simulink model "HybridStationAcceptanceTest_r1"  (R2023a)
settings: Solver=VariableStepAuto  StartTime=0.0  StopTime=240  RelTol=1e-3
libraries: simulink x43, simulink_extras x12, dspswit3 x10, spspowerguiLib x1
settings Model: PacingRate=4  Creator=jakob  LastModifiedBy=matty

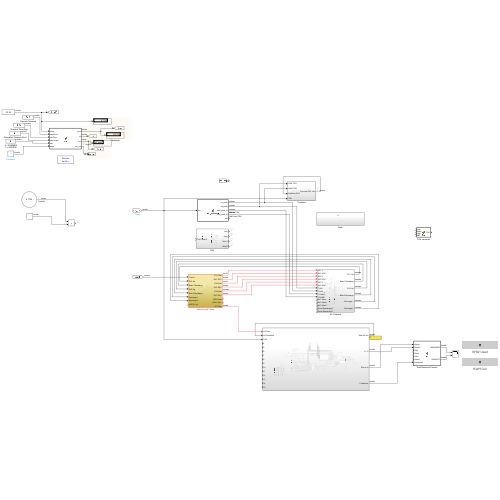
[thumbnail: Simulink's stored preview of the top-level diagram]
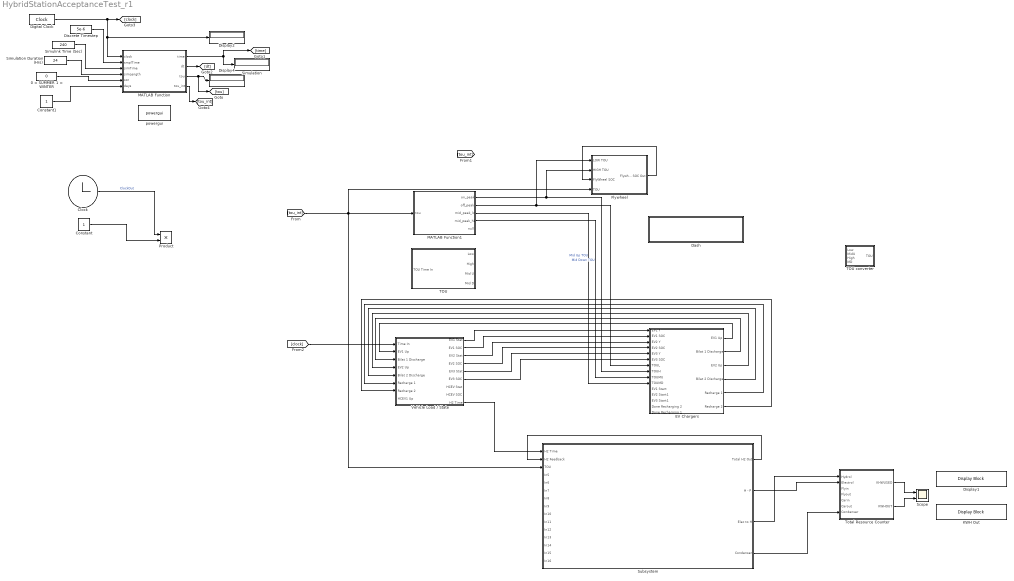
== system HybridStationAcceptanceTest_r1 ==
  0 = SUMMER 1 = WINTER : Constant  Value=0
  Clock : Clock
  Constant : Constant
  Constant1 : Constant
  Dash : Subsystem
  Digital Clock : DigitalClock  SampleTime=5e-6
  Discrete Timestep : Constant  Value=5e-6
  Display1 : DisplayBlock  LabelPosition=Hide  Transparency=1
      settings: AttributesFormatString=KHW Used
  Display2 : Display
  Display4 : Display
  EV Chargers : Subsystem
  Flywheel : Subsystem  StopFcn=CapTest
  KWH Out : DisplayBlock  LabelPosition=Hide  Transparency=1
      settings: AttributesFormatString=KWH Out
  MATLAB Function : MATLAB Function  TreatAsAtomicUnit=on
  MATLAB Function1 : MATLAB Function  TreatAsAtomicUnit=on
  Product : Product
  Scope : Scope  NumInputPorts=2
  Simulation : Display
  Simulation Duration (Hrs) : Constant  Value=24
  Simulink Time (Sec) : Constant  Value=240
  Subsystem : Subsystem
  TOU : Subsystem
  TOU converter : MATLAB Function  TreatAsAtomicUnit=on
  Total Resource Counter : MATLAB Function  TreatAsAtomicUnit=on
  Vehicle Load / State : Subsystem
  powergui : spspowerguiLib/powergui  Priority=1  SimulationMode=Discrete  SampleTime=5e-6  frequency=60  Iterations=50  frequencyindice=0  Pbase=100e6  ErrMax=1e-4  UnitsV=kV  UnitsW=MW  buscounter=0  FunctionMessages=off  echomessages=off  EnableUseOfTLC=off  CurrentSourceSwitches=off  DisableSnubberDevices=off  DisableRonSwitches=off  DisableVfSwitches=off  DisplayEquations=off  AutomaticDiscreteSolvers=off  SolverType=Tustin/Backward Euler (TBE)  Interpol=off  ExternalGateDelay=off  methode=off  Ts=100  x0status=blocks  SPID=on  SwTol=0  HookPort=off  NonlinearTolerance=1e-4  nMaxIteration=100  ContinueOnMaxIteration=off  RestoreLinks=warning  ResistiveCurrentMeasurement=off  Frange=[0:2:500]  Ylog=off  Xlog=on  ShowGrid=off  save=off  variable=ZData  structure=0  ZoomFFT=off  StartTime=0.0  cycles=1  DisplayStyle=1  fundamental=60  FreqAxis=off  MaxFrequency=1000  frequencyindicesteady=1  RmsSteady=1  display=off
  wires:
  Clock/1 -> Product/1  "ClockOut"
  Constant/1 -> Product/2
  Vehicle Load / State/1(EV1 Stat) -> EV Chargers/1(EV1 Y)
  Vehicle Load / State/2(EV1 SOC) -> EV Chargers/2(EV1 SOC)
  Vehicle Load / State/3(EV2 Stat) -> EV Chargers/3(EV2 Y)
  Vehicle Load / State/4(EV2 SOC) -> EV Chargers/4(EV2 SOC)
  Vehicle Load / State/5(EV3 Stat) -> EV Chargers/5(EV3 Y)
  Vehicle Load / State/6(EV3 SOC) -> EV Chargers/6(EV3 SOC)
  Flywheel/1(Flywheel SOC Out) -> Flywheel/3(FlyWheel SOC)
  EV Chargers/1(EV1 Up) -> Vehicle Load / State/2(EV1 Up)
  EV Chargers/2(Bilat 1 Discharge) -> Vehicle Load / State/3(Bilat 1 Discharge)
  EV Chargers/3(EV2 Up) -> Vehicle Load / State/4(EV2 Up)
  EV Chargers/4(Bilat 2 Discharge) -> Vehicle Load / State/5(Bilat 2 Discharge)
  EV Chargers/5(Recharge 1) -> Vehicle Load / State/6(Recharge 1)
  EV Chargers/6(Recharge 2) -> Vehicle Load / State/7(Recharge 2)
  Vehicle Load / State/9(H2 Time) -> Subsystem/1(H2 Time)
  Subsystem/1(Total H2 Out) -> Subsystem/2(H2 Feedback)
  Total Resource Counter/1(KHWUSED) -> Scope/1
  Total Resource Counter/2(KWHOUT) -> Scope/2
  Subsystem/4(Condenser) -> Total Resource Counter/7(Condenser)
  Subsystem/3(Elec to H) -> Total Resource Counter/1(Hydrol)
  Subsystem/2(H - P) -> Total Resource Counter/2(Electrol)
  MATLAB Function/1(time) -> [time], Simulation/1
  MATLAB Function/3(tou) -> [tou], Display4/1
  Digital Clock/1 -> [clock], MATLAB Function/1(clock), Display2/1
  Constant1/1 -> MATLAB Function/6(days)
  Discrete Timestep/1 -> MATLAB Function/2(smplTime)
  Simulink Time (Sec)/1 -> MATLAB Function/3(simTime)
  Simulation Duration (Hrs)/1 -> MATLAB Function/4(simLength)
  MATLAB Function/4(tou_int) -> [tou_int]
  MATLAB Function/2(dt) -> [dt]
  0 = SUMMER 1 = WINTER/1 -> MATLAB Function/5(szn)
  [tou_int] -> Subsystem/3(TOU), Flywheel/4(TOU), MATLAB Function1/1(tou)
  MATLAB Function1/3(mid_peak_lo) -> EV Chargers/10(TOUMD)  "Mid Up TOU"
  MATLAB Function1/1(on_peak) -> Flywheel/2(HIGH TOU), EV Chargers/8(TOUH)
  MATLAB Function1/2(off_peak) -> Flywheel/1(LOW TOU), EV Chargers/7(TOUL)
  MATLAB Function1/4(mid_peak_hi) -> EV Chargers/9(TOUMU)  "Mid Down TOU"
  [clock] -> Vehicle Load / State/1(Time In)

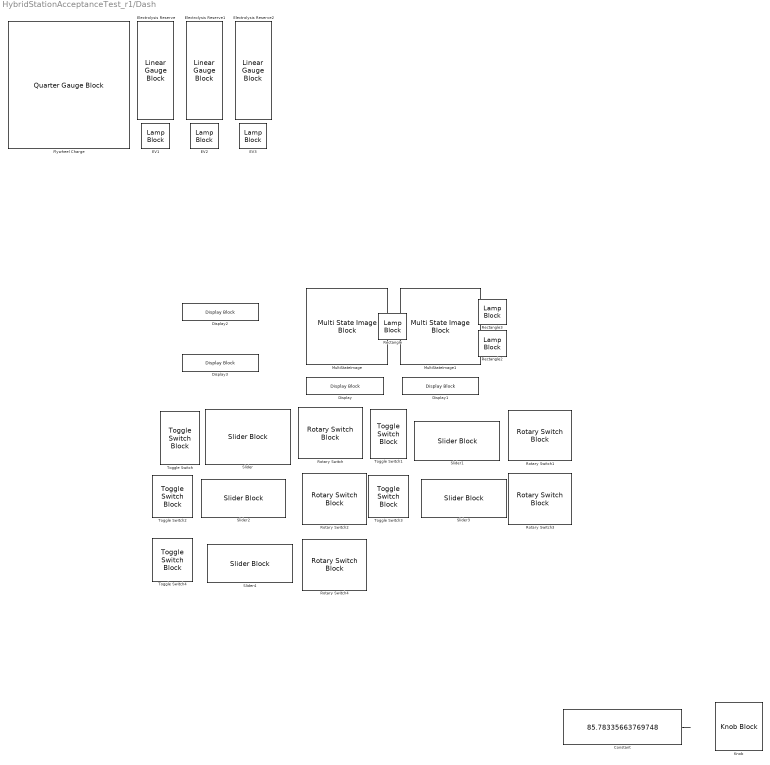
== system HybridStationAcceptanceTest_r1/Dash ==
  Constant : Constant  Value=85.78335663769748
  Display{,1..3} (4 alike) : DisplayBlock  LabelPosition=Hide  Transparency=1
      Display2 settings: AttributesFormatString=Hydrogen Output (KG)
      Display3 settings: AttributesFormatString=FCEVs Fueled
  EV1 : LampBlock  LabelPosition=Hide
  EV2 : LampBlock  LabelPosition=Hide
  EV3 : LampBlock  LabelPosition=Hide
  Electrolysis Reserve : LinearGaugeBlock  Tag=Flywheel %
  Electrolysis Reserve1 : LinearGaugeBlock  Tag=Flywheel %
  Electrolysis Reserve2 : LinearGaugeBlock  Tag=Flywheel %
  Flywheel Charge : QuarterGaugeBlock
  Knob : KnobBlock  ScaleMax=240
  MultiStateImage : MultiStateImageBlock  Description=10KG pressurized 700Bar
      settings: AttributesFormatString=10KG pressurized 700Bar
  MultiStateImage1 : MultiStateImageBlock
      settings: AttributesFormatString=10KG pressurized 200Bar
  Rectangle : LampBlock  LabelPosition=Hide  Icon=Rectangle
      settings: AttributesFormatString=Compressor
  Rectangle2 : LampBlock  LabelPosition=Hide  Icon=Rectangle
      settings: AttributesFormatString=Reverse Electrolysis
  Rectangle3 : LampBlock  LabelPosition=Hide  Icon=Rectangle
      settings: AttributesFormatString=Electrolysis
  Rotary Switch{,1..4} (5 alike) : RotarySwitchBlock
      settings: Values={{'>0', '1', '2', '3', '4'}, [0 1 2 3 4]}
      settings: AttributesFormatString=Hydrogren Level
  Slider{,1..4} (5 alike) : SliderBlock  ScaleMax=240
      settings: AttributesFormatString=Start Time
  Toggle Switch{,1..4} (5 alike) : ToggleSwitchBlock
      settings: Values={{'Off', 'On'}, [0 1]}
  wires:
  Constant/1 -> ?

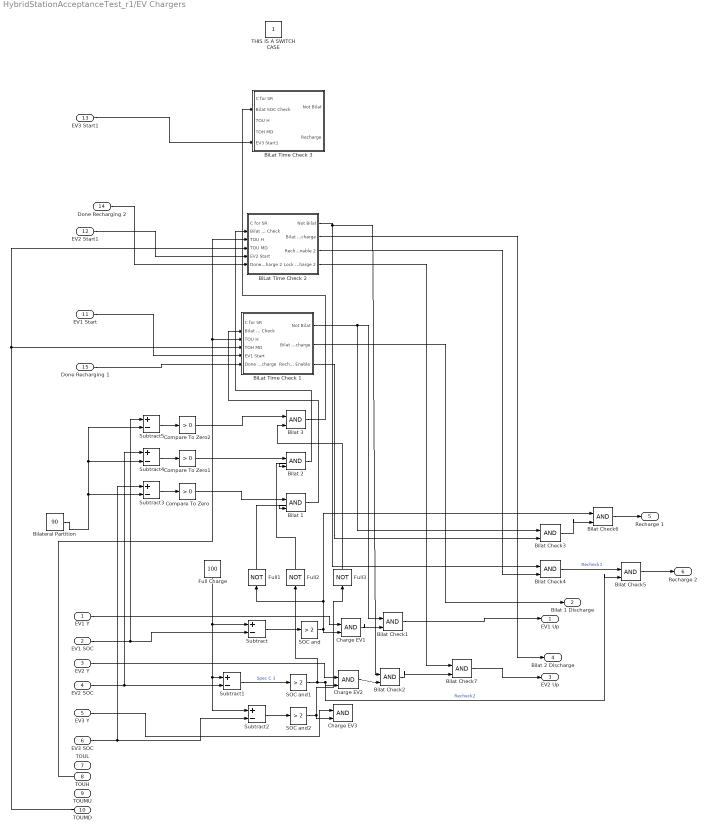
== system HybridStationAcceptanceTest_r1/EV Chargers ==
  EV1 Y : Inport
  EV1 SOC : Inport  Port=2
  EV2 Y : Inport  Port=3
  EV2 SOC : Inport  Port=4
  EV3 Y : Inport  Port=5
  EV3 SOC : Inport  Port=6
  TOUL : Inport  Port=7
  TOUH : Inport  Port=8
  TOUMU : Inport  Port=9
  TOUMD : Inport  Port=10
  EV1 Start : Inport  Port=11
  EV2 Start1 : Inport  Port=12
  EV3 Start1 : Inport  Port=13
  Done Recharging 2 : Inport  Port=14
  Done Recharging 1 : Inport  Port=15
  BiLat Time Check 1 : Subsystem
  BiLat Time Check 2 : Subsystem
  BiLat Time Check 3 : Subsystem
  Bilat 1 : Logic  IconShape=distinctive  AllPortsSameDT=off  OutDataTypeStr=boolean
  Bilat 2 : Logic  IconShape=distinctive  AllPortsSameDT=off  OutDataTypeStr=boolean
  Bilat 3 : Logic  IconShape=distinctive  AllPortsSameDT=off  OutDataTypeStr=boolean
  Bilat Check{1..7} (7 alike) : Logic  IconShape=distinctive  AllPortsSameDT=off  OutDataTypeStr=boolean
  Bilateral Partition : Constant  Value=90
  Charge EV1 : Logic  IconShape=distinctive  AllPortsSameDT=off  OutDataTypeStr=boolean
  Charge EV2 : Logic  IconShape=distinctive  AllPortsSameDT=off  OutDataTypeStr=boolean
  Charge EV3 : Logic  IconShape=distinctive  AllPortsSameDT=off  OutDataTypeStr=boolean
  Compare To Zero : simulink/Logic and Bit Operations/Compare To Zero  relop=>  OutDataTypeStr=boolean
  Compare To Zero1 : simulink/Logic and Bit Operations/Compare To Zero  relop=>  OutDataTypeStr=boolean
  Compare To Zero2 : simulink/Logic and Bit Operations/Compare To Zero  relop=>  OutDataTypeStr=boolean
  Full Charge : Constant  Value=100
  Full1 : Logic  Operator=NOT  IconShape=distinctive  AllPortsSameDT=off  OutDataTypeStr=boolean
  Full2 : Logic  Operator=NOT  IconShape=distinctive  AllPortsSameDT=off  OutDataTypeStr=boolean
  Full3 : Logic  Operator=NOT  IconShape=distinctive  AllPortsSameDT=off  OutDataTypeStr=boolean
  SOC and : simulink/Logic and Bit Operations/Compare To Constant  relop=>  const=2  OutDataTypeStr=boolean
  SOC and1 : simulink/Logic and Bit Operations/Compare To Constant  relop=>  const=2  OutDataTypeStr=boolean
  SOC and2 : simulink/Logic and Bit Operations/Compare To Constant  relop=>  const=2  OutDataTypeStr=boolean
  Subtract{,1..5} (6 alike) : Sum  Inputs=+-
  THIS IS A SWITCH CASE : Constant
  EV1 Up : Outport
  Bilat 1 Discharge : Outport  Port=2
  EV2 Up : Outport  Port=3
  Bilat 2 Discharge : Outport  Port=4
  Recharge 1 : Outport  Port=5
  Recharge 2 : Outport  Port=6
  wires:
  Full Charge/1 -> Subtract2/1, Subtract1/1, Subtract/1
  EV1 SOC/1 -> Subtract5/1, Subtract/2
  EV2 Y/1 -> Charge EV2/1
  SOC and1/1 -> Bilat Check5/2, Charge EV2/2, Full2/1  "Recheck2"
  Subtract1/1 -> SOC and1/1  "Spec C 3"
  SOC and2/1 -> Full3/1, Charge EV3/2
  SOC and/1 -> Bilat Check6/1, Full1/1, Charge EV1/2
  Subtract/1 -> SOC and/1
  Subtract2/1 -> SOC and2/1
  EV3 SOC/1 -> Subtract3/1, Subtract2/2
  Charge EV2/1 -> Bilat Check2/2
  EV1 Y/1 -> Charge EV1/1
  EV3 Y/1 -> Charge EV3/1
  EV2 SOC/1 -> Subtract4/1, Subtract1/2
  Subtract3/1 -> Compare To Zero/1
  Subtract4/1 -> Compare To Zero1/1
  Subtract5/1 -> Compare To Zero2/1
  Full1/1 -> Bilat 1/2
  Compare To Zero/1 -> Bilat 1/1
  Compare To Zero1/1 -> Bilat 2/1
  Compare To Zero2/1 -> Bilat 3/1
  Full2/1 -> Bilat 2/2
  Full3/1 -> Bilat 3/2
  Bilateral Partition/1 -> Subtract4/2, Subtract5/2, Subtract3/2
  Bilat 3/1 -> BiLat Time Check 3/2(Bilat SOC Check)
  Bilat 2/1 -> BiLat Time Check 2/2(Bilat SOC Check)
  EV1 Start/1 -> BiLat Time Check 1/5(EV1 Start)
  Bilat 1/1 -> BiLat Time Check 1/2(Bilat SOC Check)
  TOUH/1 -> BiLat Time Check 2/3(TOU H), BiLat Time Check 1/3(TOU H)
  TOUMD/1 -> BiLat Time Check 2/4(TOU MD), BiLat Time Check 1/4(TOH MD)
  BiLat Time Check 1/2(Bilat Discharge) -> Bilat 1 Discharge/1
  BiLat Time Check 1/1(Not Bilat) -> Bilat Check3/1, Bilat Check1/1
  Charge EV1/1 -> Bilat Check1/2
  EV2 Start1/1 -> BiLat Time Check 2/5(EV2 Start)
  EV3 Start1/1 -> BiLat Time Check 3/5(EV3 Start1)
  BiLat Time Check 2/1(Not Bilat) -> Bilat Check4/1, Bilat Check2/1
  BiLat Time Check 2/2(Bilat Discharge) -> Bilat 2 Discharge/1
  Bilat Check2/1 -> Bilat Check7/2
  Bilat Check1/1 -> EV1 Up/1
  BiLat Time Check 1/3(Recharge Enable) -> Bilat Check3/2
  BiLat Time Check 2/3(Recharge Enable 2) -> Bilat Check4/2
  Done Recharging 2/1 -> BiLat Time Check 2/6(Done Recharge 2)
  Done Recharging 1/1 -> BiLat Time Check 1/6(Done Recharge)
  Bilat Check3/1 -> Bilat Check6/2
  Bilat Check4/1 -> Bilat Check5/1  "Recheck1"
  Bilat Check5/1 -> Recharge 2/1
  Bilat Check6/1 -> Recharge 1/1
  Bilat Check7/1 -> EV2 Up/1
  BiLat Time Check 2/4(Lock Out Recharge 2) -> Bilat Check7/1

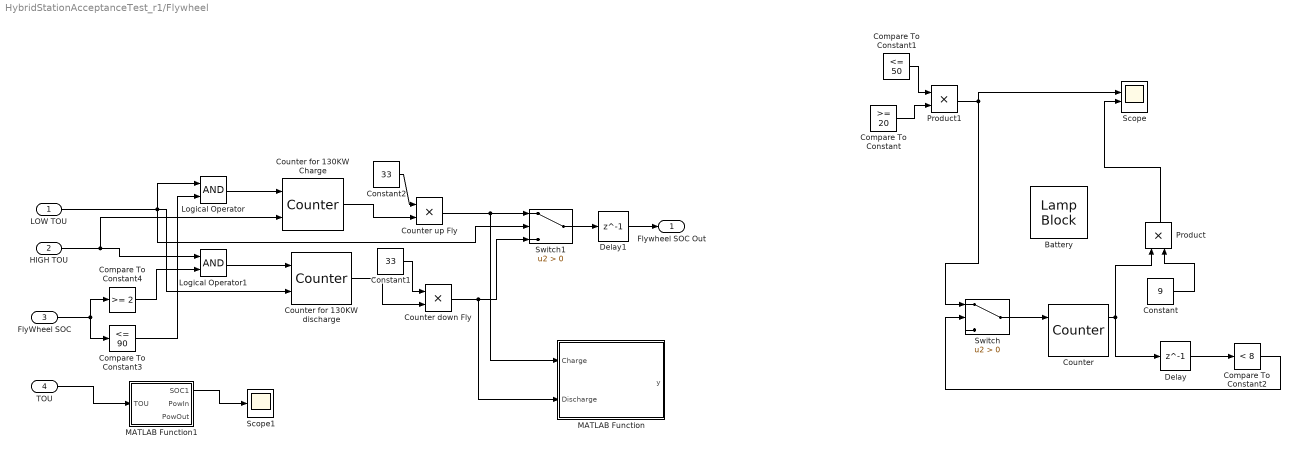
== system HybridStationAcceptanceTest_r1/Flywheel ==
  LOW TOU : Inport
  HIGH TOU : Inport  Port=2
  FlyWheel SOC : Inport  Port=3
  TOU : Inport  Port=4
  Battery : LampBlock  LabelPosition=Hide  Icon=Battery
  Compare To Constant : simulink/Logic and Bit Operations/Compare To Constant  relop=>=  const=20  OutDataTypeStr=boolean
  Compare To Constant1 : simulink/Logic and Bit Operations/Compare To Constant  relop=<=  const=50  OutDataTypeStr=boolean
  Compare To Constant2 : simulink/Logic and Bit Operations/Compare To Constant  relop=<  const=8  OutDataTypeStr=boolean
  Compare To Constant3 : simulink/Logic and Bit Operations/Compare To Constant  relop=<=  const=90  OutDataTypeStr=boolean
  Compare To Constant4 : simulink/Logic and Bit Operations/Compare To Constant  relop=>=  const=2  OutDataTypeStr=boolean
  Constant : Constant  Value=9
  Constant1 : Constant  Value=33
  Constant2 : Constant  Value=33
  Counter : dspswit3/Counter  Direction=Up  CountEvent=Non-zero sample  CounterSize=User defined  MaxCount=100  InitialCount=0  Output=Count and Hit  HitValue=32  ResetInput=on  SamplesPerFrame=1  Ts=1  CntDtype=single  HitDtype=Logical
  Counter down Fly : Product
  Counter for 130KW Charge : dspswit3/Counter  Direction=Up  CountEvent=Non-zero sample  CounterSize=User defined  MaxCount=3  InitialCount=0  Output=Count  HitValue=32  ResetInput=on  SamplesPerFrame=1  Ts=1  CntDtype=single  HitDtype=Logical
  Counter for 130KW discharge : dspswit3/Counter  Direction=Down  CountEvent=Non-zero sample  CounterSize=User defined  MaxCount=10  InitialCount=3  Output=Count  HitValue=32  ResetInput=on  SamplesPerFrame=1  Ts=1  CntDtype=single  HitDtype=Logical
  Counter up Fly : Product
  Delay : Delay  DelayLength=1  InitialCondition=0
  Delay1 : Delay  DelayLength=1  InitialCondition=0
  Logical Operator : Logic  AllPortsSameDT=off  OutDataTypeStr=boolean
  Logical Operator1 : Logic  AllPortsSameDT=off  OutDataTypeStr=boolean
  MATLAB Function : MATLAB Function  TreatAsAtomicUnit=on
  MATLAB Function1 : MATLAB Function  TreatAsAtomicUnit=on
  Product : Product
  Product1 : Product
  Scope : Scope  NumInputPorts=4
  Scope1 : Scope
  Switch : Switch  Criteria=u2 > Threshold  SaturateOnIntegerOverflow=off  InputSameDT=off
  Switch1 : Switch  Criteria=u2 > Threshold  SaturateOnIntegerOverflow=off  InputSameDT=off
  Flywheel SOC Out : Outport
  wires:
  Compare To Constant1/1 -> Product1/1
  Compare To Constant/1 -> Product1/2
  Counter/1 -> Product/1, Delay/1
  Product1/1 -> Switch/1, Scope/2
  Switch/1 -> Counter/1
  Compare To Constant2/1 -> Switch/2
  Delay/1 -> Compare To Constant2/1
  Constant/1 -> Product/2
  Product/1 -> Scope/3
  LOW TOU/1 -> Counter for 130KW discharge/2, Logical Operator/1, Switch1/2
  FlyWheel SOC/1 -> Compare To Constant4/1, Compare To Constant3/1
  Compare To Constant3/1 -> Logical Operator/2
  Compare To Constant4/1 -> Logical Operator1/2
  HIGH TOU/1 -> Counter for 130KW Charge/2, Logical Operator1/1
  Logical Operator1/1 -> Counter for 130KW discharge/1
  Constant1/1 -> Counter down Fly/1
  Counter for 130KW discharge/1 -> Counter down Fly/2
  Counter down Fly/1 -> MATLAB Function/2(Discharge), Switch1/3
  Constant2/1 -> Counter up Fly/1
  Counter for 130KW Charge/1 -> Counter up Fly/2
  Logical Operator/1 -> Counter for 130KW Charge/1
  Counter up Fly/1 -> MATLAB Function/1(Charge), Switch1/1
  Switch1/1 -> Delay1/1
  Delay1/1 -> Flywheel SOC Out/1
  TOU/1 -> MATLAB Function1/1(TOU)
  MATLAB Function1/1(SOC1) -> Scope1/1

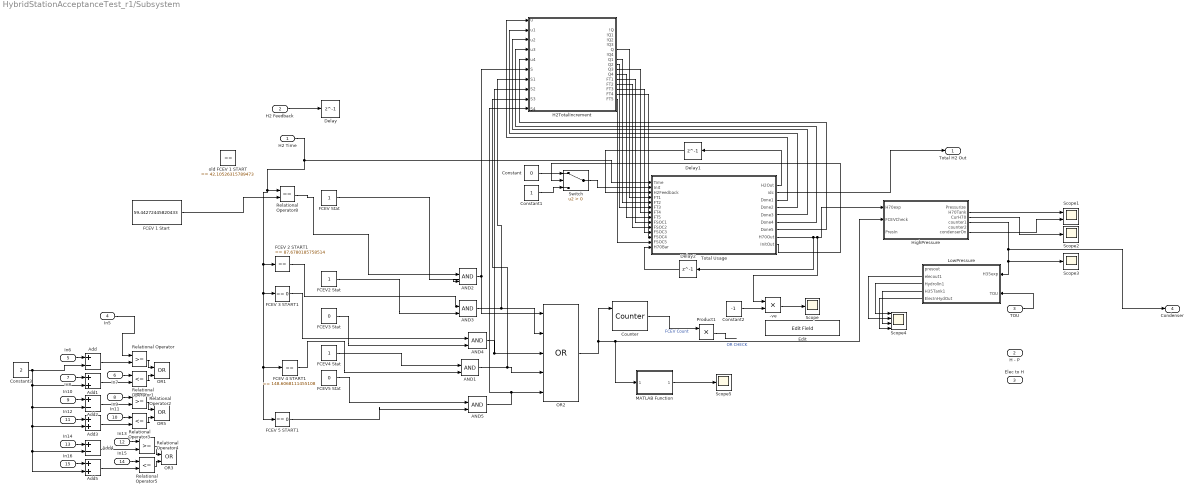
== system HybridStationAcceptanceTest_r1/Subsystem ==
  H2 Time : Inport
  H2 Feedback : Inport  Port=2
  TOU : Inport  Port=3
  In5 : Inport  Port=4
  In6 : Inport  Port=5
  In7 : Inport  Port=6
  In8 : Inport  Port=7
  In9 : Inport  Port=8
  In10 : Inport  Port=9
  In11 : Inport  Port=10
  In12 : Inport  Port=11
  In13 : Inport  Port=12
  In14 : Inport  Port=13
  In15 : Inport  Port=14
  In16 : Inport  Port=15
  " FCEV 3 START1" : simulink/Logic and Bit Operations/Compare To Constant  relop===  const=0  OutDataTypeStr=boolean
  " FCEV 5 START1" : simulink/Logic and Bit Operations/Compare To Constant  relop===  const=0  OutDataTypeStr=boolean
  -ve : Product
  AND{1..5} (5 alike) : Logic  IconShape=distinctive  AllPortsSameDT=off  OutDataTypeStr=boolean
  Add : Sum  Inputs=+-
  Add1 : Sum
  Add2 : Sum  Inputs=+-
  Add3 : Sum
  Add4 : Sum  Inputs=+-
  Add5 : Sum
  Constant : Constant  Value=0
  Constant1 : Constant
  Constant2 : Constant  Value=-1
  Constant3 : Constant  Value=2
  Counter : dspswit3/Counter  Direction=Up  CountEvent=Rising edge  CounterSize=User defined  MaxCount=255  InitialCount=0  Output=Count  HitValue=32  ResetInput=on  SamplesPerFrame=1  Ts=1  CntDtype=double  HitDtype=Logical
  Delay : Delay  DelayLength=1  InitialCondition=0
  Delay1 : Delay  DelayLength=1  InitialCondition=0
  Delay2 : Delay  DelayLength=1  InitialCondition=0
  Edit : EditField  LabelPosition=Hide  ShowInitialText=on  Alignment=Center
  FCEV 1 Start : Constant  Value=59.44272445820433
  FCEV 2 START1 : simulink/Logic and Bit Operations/Compare To Constant  relop===  const=87.6780185758514  OutDataTypeStr=boolean
      settings: AttributesFormatString=FCEV2
  FCEV 4 START1 : simulink/Logic and Bit Operations/Compare To Constant  relop===  const=148.6068111455108  OutDataTypeStr=boolean
      settings: AttributesFormatString=FCEV2
  FCEV Stat : Constant
  FCEV2 Stat : Constant
  FCEV3 Stat : Constant  Value=0
  FCEV4 Stat : Constant
  FCEV5 Stat : Constant  Value=0
  H2TotalIncrement : Subsystem
  HighPressure : MATLAB Function  TreatAsAtomicUnit=on
  LowPressure : MATLAB Function  TreatAsAtomicUnit=on
  MATLAB Function : MATLAB Function  TreatAsAtomicUnit=on
  OR1 : Logic  Operator=OR  IconShape=distinctive  AllPortsSameDT=off  OutDataTypeStr=boolean
  OR2 : Logic  Operator=OR  Inputs=5  IconShape=distinctive  AllPortsSameDT=off  OutDataTypeStr=boolean
  OR3 : Logic  Operator=OR  IconShape=distinctive  AllPortsSameDT=off  OutDataTypeStr=boolean
  OR5 : Logic  Operator=OR  IconShape=distinctive  AllPortsSameDT=off  OutDataTypeStr=boolean
  Product1 : Product
  Relational Operator : RelationalOperator  OutDataTypeStr=boolean  RndMeth=Simplest  InputSameDT=off
  Relational Operator1 : RelationalOperator  Operator=<=  OutDataTypeStr=boolean  RndMeth=Simplest  InputSameDT=off
  Relational Operator2 : RelationalOperator  OutDataTypeStr=boolean  RndMeth=Simplest  InputSameDT=off
  Relational Operator3 : RelationalOperator  Operator=<=  OutDataTypeStr=boolean  RndMeth=Simplest  InputSameDT=off
  Relational Operator4 : RelationalOperator  OutDataTypeStr=boolean  RndMeth=Simplest  InputSameDT=off
  Relational Operator5 : RelationalOperator  Operator=<=  OutDataTypeStr=boolean  RndMeth=Simplest  InputSameDT=off
  Relational Operator8 : RelationalOperator  Operator===  OutDataTypeStr=boolean  RndMeth=Simplest  InputSameDT=off
  Scope{,2..3,5} (4 alike) : Scope
  Scope1 : Scope  NumInputPorts=2
  Scope4 : Scope  NumInputPorts=4
  Switch : Switch  Criteria=u2 > Threshold  SaturateOnIntegerOverflow=off  InputSameDT=off
  Total Usage : MATLAB Function  TreatAsAtomicUnit=on
  old FCEV 1 START : simulink/Logic and Bit Operations/Compare To Constant  relop===  const=42.10526315789473  OutDataTypeStr=boolean
  Total H2 Out : Outport
  H - P : Outport  Port=2
  Elec to H : Outport  Port=3
  Condenser : Outport  Port=4
  wires:
  Add4/1 -> Relational Operator4/2
  Relational Operator2/1 -> OR5/1
  Relational Operator3/1 -> OR5/2
  AND2/1 -> H2TotalIncrement/6(S), OR2/1
  Add/1 -> Relational Operator/2
  In8/1 -> Add1/1
  Add3/1 -> Relational Operator3/2
  Relational Operator1/1 -> OR1/2
  Constant3/1 -> Add5/2, Add4/2, Add3/2, Add2/2, Add1/2, Add/2
  Product1/1 -> ?
  In12/1 -> Add3/1
  In7/1 -> Relational Operator1/1
  " FCEV 3 START1"/1 -> AND4/1
  In14/1 -> Add4/1
  Relational Operator5/1 -> OR3/2
  OR2/1 -> MATLAB Function/1(FCEVIn), HighPressure/2(FCEVCheck), Counter/1  "OR CHECK"
  H2 Time/1 -> Total Usage/1(Time), Relational Operator8/1, " FCEV 5 START1"/1, FCEV 4 START1/1, " FCEV 3 START1"/1, FCEV 2 START1/1
  In13/1 -> Relational Operator4/1
  Relational Operator/1 -> OR1/1
  Add2/1 -> Relational Operator2/2
  In10/1 -> Add2/1
  In11/1 -> Relational Operator3/1
  FCEV 2 START1/1 -> AND3/1
  Add1/1 -> Relational Operator1/2
  AND4/1 -> OR2/3, H2TotalIncrement/8(S2)
  FCEV3 Stat/1 -> AND4/2
  In15/1 -> Relational Operator5/1
  AND3/1 -> H2TotalIncrement/7(S1), OR2/2
  In9/1 -> Relational Operator2/1
  FCEV Stat/1 -> AND2/2
  FCEV2 Stat/1 -> AND3/2
  Counter/1 -> Product1/1  "FCEV Count"
  Add5/1 -> Relational Operator5/2
  Relational Operator4/1 -> OR3/1
  In6/1 -> Add/1
  In16/1 -> Add5/1
  In5/1 -> Relational Operator/1
  Relational Operator8/1 -> AND2/1
  H2 Feedback/1 -> Delay/1
  FCEV 1 Start/1 -> Relational Operator8/2
  Total Usage/1(H2Out) -> Delay1/1
  Total Usage/2(idc) -> Total H2 Out/1
  AND1/1 -> OR2/4, H2TotalIncrement/9(S3)
  AND5/1 -> H2TotalIncrement/10(S4), OR2/5
  FCEV5 Stat/1 -> AND5/1
  " FCEV 5 START1"/1 -> AND5/2
  FCEV4 Stat/1 -> AND1/1
  FCEV 4 START1/1 -> AND1/2
  Total Usage/3(Done1) -> H2TotalIncrement/1(u)
  Total Usage/4(Done2) -> H2TotalIncrement/2(u1)
  Total Usage/5(Done3) -> H2TotalIncrement/3(u2)
  Total Usage/6(Done4) -> H2TotalIncrement/4(u3)
  Total Usage/7(Done5) -> H2TotalIncrement/5(u4)
  Total Usage/8(H70Out) -> -ve/1, HighPressure/1(H70exp), Delay2/1
  Constant1/1 -> Switch/3
  Constant/1 -> Switch/1
  Total Usage/9(InitOut) -> Switch/2
  H2TotalIncrement/5(Q) -> Total Usage/4(FT1)
  H2TotalIncrement/7(Q1) -> Total Usage/5(FT2)
  H2TotalIncrement/8(Q2) -> Total Usage/6(FT3)
  H2TotalIncrement/9(Q3) -> Total Usage/7(FT4)
  H2TotalIncrement/10(Q4) -> Total Usage/8(FT5)
  Delay2/1 -> Total Usage/14(H70Bar)
  H2TotalIncrement/11(FT1) -> Total Usage/9(FSOC1)
  H2TotalIncrement/12(FT2) -> Total Usage/10(FSOC2)
  H2TotalIncrement/13(FT3) -> Total Usage/11(FSOC3)
  H2TotalIncrement/14(FT4) -> Total Usage/12(FSOC4)
  H2TotalIncrement/15(FT5) -> Total Usage/13(FSOC5)
  Delay1/1 -> Total Usage/3(H2Feedback)
  Switch/1 -> Total Usage/2(Init)
  Constant2/1 -> -ve/2
  -ve/1 -> Scope/1
  HighPressure/2(H70Tank) -> Scope1/1
  HighPressure/3(CurH70) -> Scope2/1
  HighPressure/4(counter1) -> Condenser/1, LowPressure/1(H35exp), Scope3/1
  TOU/1 -> LowPressure/2(TOU)
  LowPressure/3(HydrolIn1) -> Scope4/1
  LowPressure/2(elecout1) -> Scope4/2
  LowPressure/4(H35Tank1) -> Scope4/3
  LowPressure/5(ElecInHydOut) -> Scope4/4
  HighPressure/6(condenserOn) -> Scope1/2
  MATLAB Function/1(FCEVPres) -> Scope5/1

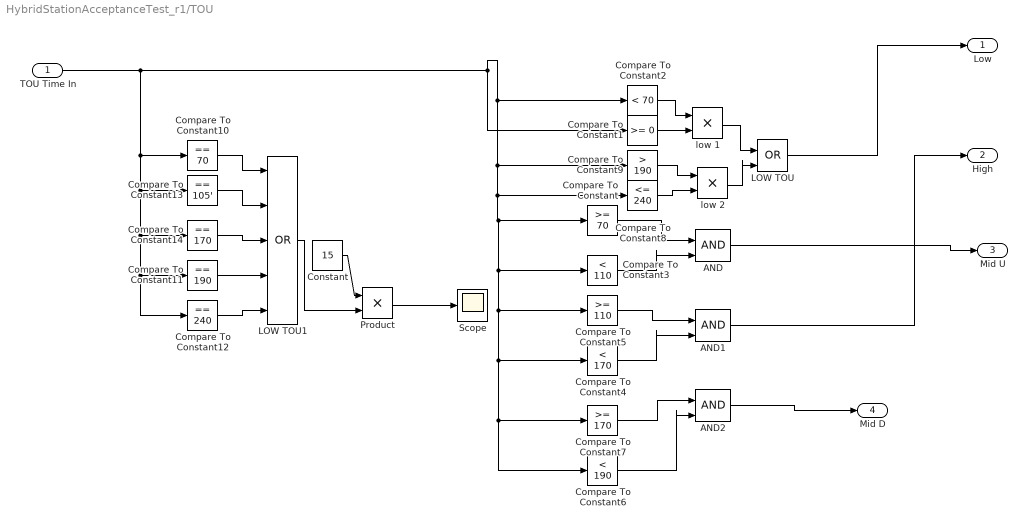
== system HybridStationAcceptanceTest_r1/TOU ==
  TOU Time In : Inport
  AND : Logic  IconShape=distinctive  AllPortsSameDT=off  OutDataTypeStr=boolean
  AND1 : Logic  IconShape=distinctive  AllPortsSameDT=off  OutDataTypeStr=boolean
  AND2 : Logic  IconShape=distinctive  AllPortsSameDT=off  OutDataTypeStr=boolean
  Compare To Constant : simulink/Logic and Bit Operations/Compare To Constant  relop=>=  const=70  OutDataTypeStr=boolean
  Compare To Constant1 : simulink/Logic and Bit Operations/Compare To Constant  relop=>=  const=0  OutDataTypeStr=boolean
  Compare To Constant10 : simulink/Logic and Bit Operations/Compare To Constant  relop===  const=70  OutDataTypeStr=boolean
  Compare To Constant11 : simulink/Logic and Bit Operations/Compare To Constant  relop===  const=190  OutDataTypeStr=boolean
  Compare To Constant12 : simulink/Logic and Bit Operations/Compare To Constant  relop===  const=240  OutDataTypeStr=boolean
  Compare To Constant13 : simulink/Logic and Bit Operations/Compare To Constant  relop===  const=105'  OutDataTypeStr=boolean
  Compare To Constant14 : simulink/Logic and Bit Operations/Compare To Constant  relop===  const=170  OutDataTypeStr=boolean
  Compare To Constant2 : simulink/Logic and Bit Operations/Compare To Constant  relop=<  const=70  OutDataTypeStr=boolean
  Compare To Constant3 : simulink/Logic and Bit Operations/Compare To Constant  relop=<  const=110  OutDataTypeStr=boolean
  Compare To Constant4 : simulink/Logic and Bit Operations/Compare To Constant  relop=<  const=170  OutDataTypeStr=boolean
  Compare To Constant5 : simulink/Logic and Bit Operations/Compare To Constant  relop=>=  const=110  OutDataTypeStr=boolean
  Compare To Constant6 : simulink/Logic and Bit Operations/Compare To Constant  relop=<  const=190  OutDataTypeStr=boolean
  Compare To Constant7 : simulink/Logic and Bit Operations/Compare To Constant  relop=>=  const=170  OutDataTypeStr=boolean
  Compare To Constant8 : simulink/Logic and Bit Operations/Compare To Constant  relop=<=  const=240  OutDataTypeStr=boolean
  Compare To Constant9 : simulink/Logic and Bit Operations/Compare To Constant  relop=>  const=190  OutDataTypeStr=boolean
  Constant : Constant  Value=15
  LOW TOU : Logic  Operator=OR  IconShape=distinctive  AllPortsSameDT=off  OutDataTypeStr=boolean
  LOW TOU1 : Logic  Operator=OR  Inputs=5  IconShape=distinctive  AllPortsSameDT=off  OutDataTypeStr=boolean
  Product : Product
  Scope : Scope
  low 1 : Product
  low 2 : Product
  Low : Outport
  High : Outport  Port=2
  Mid U : Outport  Port=3
  Mid D : Outport  Port=4
  wires:
  Compare To Constant6/1 -> AND2/2
  Compare To Constant/1 -> AND/1
  low 2/1 -> LOW TOU/2
  Compare To Constant5/1 -> AND1/1
  Compare To Constant8/1 -> low 2/2
  TOU Time In/1 -> Compare To Constant12/1, Compare To Constant11/1, Compare To Constant14/1, Compare To Constant13/1, Compare To Constant10/1, Compare To Constant9/1, Compare To Constant8/1, Compare To Constant6/1, Compare To Constant7/1, Compare To Constant4/1, Compare To Constant5/1, Compare To Constant3/1, Compare To Constant/1, Compare To Constant2/1, Compare To Constant1/1
  Compare To Constant3/1 -> AND/2
  AND1/1 -> High/1
  Compare To Constant2/1 -> low 1/1
  Compare To Constant1/1 -> low 1/2
  Compare To Constant7/1 -> AND2/1
  Compare To Constant4/1 -> AND1/2
  AND/1 -> Mid U/1
  Compare To Constant9/1 -> low 2/1
  low 1/1 -> LOW TOU/1
  LOW TOU/1 -> Low/1
  AND2/1 -> Mid D/1
  Constant/1 -> Product/1
  LOW TOU1/1 -> Product/2
  Product/1 -> Scope/1
  Compare To Constant10/1 -> LOW TOU1/1
  Compare To Constant13/1 -> LOW TOU1/2
  Compare To Constant14/1 -> LOW TOU1/3
  Compare To Constant11/1 -> LOW TOU1/4
  Compare To Constant12/1 -> LOW TOU1/5

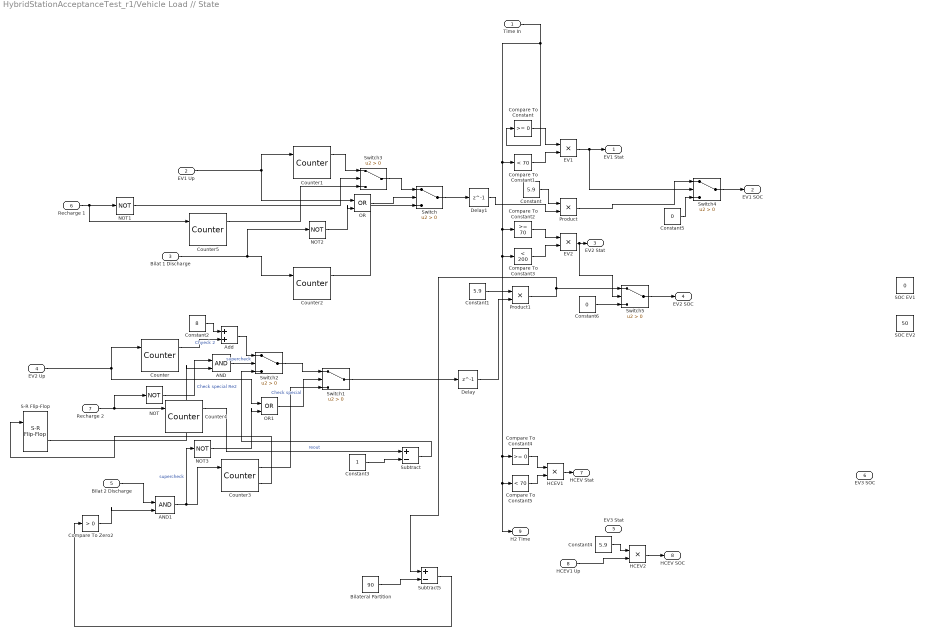
== system HybridStationAcceptanceTest_r1/Vehicle Load // State ==
  Time In : Inport
  EV1 Up : Inport  Port=2
  Bilat 1 Discharge : Inport  Port=3
  EV2 Up : Inport  Port=4
  Bilat 2 Discharge : Inport  Port=5
  Recharge 1 : Inport  Port=6
  Recharge 2 : Inport  Port=7
  HCEV1 Up : Inport  Port=8
  AND : Logic  IconShape=distinctive  AllPortsSameDT=off  OutDataTypeStr=boolean
  AND1 : Logic  IconShape=distinctive  AllPortsSameDT=off  OutDataTypeStr=boolean
  Add : Sum
  Bilateral Partition : Constant  Value=90
  Compare To Constant : simulink/Logic and Bit Operations/Compare To Constant  relop=>=  const=0  OutDataTypeStr=boolean
  Compare To Constant1 : simulink/Logic and Bit Operations/Compare To Constant  relop=<  const=70  OutDataTypeStr=boolean
  Compare To Constant2 : simulink/Logic and Bit Operations/Compare To Constant  relop=>=  const=70  OutDataTypeStr=boolean
  Compare To Constant3 : simulink/Logic and Bit Operations/Compare To Constant  relop=<  const=200  OutDataTypeStr=boolean
  Compare To Constant4 : simulink/Logic and Bit Operations/Compare To Constant  relop=>=  const=0  OutDataTypeStr=boolean
  Compare To Constant5 : simulink/Logic and Bit Operations/Compare To Constant  relop=<  const=70  OutDataTypeStr=boolean
  Compare To Zero2 : simulink/Logic and Bit Operations/Compare To Zero  relop=>  OutDataTypeStr=boolean
  Constant : Constant  Value=5.9
  Constant1 : Constant  Value=5.9
  Constant2 : Constant  Value=8
  Constant3 : Constant
  Constant4 : Constant  Value=5.9
  Constant5 : Constant  Value=0
  Constant6 : Constant  Value=0
  Counter : dspswit3/Counter  Direction=Up  CountEvent=Non-zero sample  CounterSize=User defined  MaxCount=17  InitialCount=0  Output=Count and Hit  HitValue=9  ResetInput=on  SamplesPerFrame=1  Ts=1  CntDtype=single  HitDtype=Logical
  Counter1 : dspswit3/Counter  Direction=Up  CountEvent=Non-zero sample  CounterSize=User defined  MaxCount=100  InitialCount=0  Output=Count and Hit  HitValue=32  ResetInput=on  SamplesPerFrame=1  Ts=1  CntDtype=single  HitDtype=Logical
  Counter2 : dspswit3/Counter  Direction=Down  CountEvent=Non-zero sample  CounterSize=User defined  MaxCount=100  InitialCount=17  Output=Count and Hit  HitValue=32  ResetInput=on  SamplesPerFrame=1  Ts=1  CntDtype=single  HitDtype=Logical
  Counter3 : dspswit3/Counter  Direction=Down  CountEvent=Non-zero sample  CounterSize=User defined  MaxCount=17  InitialCount=17  Output=Count and Hit  HitValue=15  ResetInput=on  SamplesPerFrame=1  Ts=1  CntDtype=single  HitDtype=Logical
  Counter4 : dspswit3/Counter  Direction=Up  CountEvent=Non-zero sample  CounterSize=User defined  MaxCount=18  InitialCount=15  Output=Count and Hit  HitValue=100  ResetInput=on  SamplesPerFrame=1  Ts=1  CntDtype=single  HitDtype=Logical
  Counter5 : dspswit3/Counter  Direction=Up  CountEvent=Non-zero sample  CounterSize=User defined  MaxCount=100  InitialCount=15  Output=Count and Hit  HitValue=32  ResetInput=on  SamplesPerFrame=1  Ts=1  CntDtype=single  HitDtype=Logical
  Delay : Delay  DelayLength=1  InitialCondition=0
  Delay1 : Delay  DelayLength=1  InitialCondition=0
  EV1 : Product
  EV2 : Product
  HCEV1 : Product
  HCEV2 : Product
  NOT{,1..3} (4 alike) : Logic  Operator=NOT  IconShape=distinctive  AllPortsSameDT=off  OutDataTypeStr=boolean
  OR : Logic  Operator=OR  IconShape=distinctive  AllPortsSameDT=off  OutDataTypeStr=boolean
  OR1 : Logic  Operator=OR  IconShape=distinctive  AllPortsSameDT=off  OutDataTypeStr=boolean
  Product : Product
  Product1 : Product
  S-R Flip-Flop : simulink_extras/Flip Flops/S-R Flip-Flop  initial_condition=0
  SOC EV1 : Constant  Value=0
  SOC EV2 : Constant  Value=50
  Subtract : Sum  Inputs=+-
  Subtract5 : Sum  Inputs=+-
  Switch{,1..5} (6 alike) : Switch  Criteria=u2 > Threshold  SaturateOnIntegerOverflow=off  InputSameDT=off
  EV1 Stat : Outport
  EV1 SOC : Outport  Port=2
  EV2 Stat : Outport  Port=3
  EV2 SOC : Outport  Port=4
  EV3 Stat : Outport  Port=5
  EV3 SOC : Outport  Port=6
  HCEV Stat : Outport  Port=7
  HCEV SOC : Outport  Port=8
  H2 Time : Outport  Port=9
  wires:
  Time In/1 -> H2 Time/1, Compare To Constant5/1, Compare To Constant4/1, Compare To Constant3/1, Compare To Constant2/1, Compare To Constant1/1, Compare To Constant/1
  Compare To Constant3/1 -> EV2/2
  Compare To Constant2/1 -> EV2/1
  Compare To Constant/1 -> EV1/1
  Compare To Constant1/1 -> EV1/2
  HCEV1/1 -> HCEV Stat/1
  EV2 Up/1 -> OR1/1, Counter/1
  EV1 Up/1 -> OR/1, Counter1/1
  Bilat 1 Discharge/1 -> NOT2/1, Counter2/1
  Switch/1 -> Delay1/1
  Counter2/1 -> Switch/3
  Switch1/1 -> Delay/1
  Switch2/1 -> Switch1/1
  Counter/1 -> Add/2  "Chyeck 2"
  Recharge 2/1 -> NOT/1, Counter4/1
  NOT/1 -> AND/1  "Check special Re2"
  Counter5/1 -> Switch3/3
  Recharge 1/1 -> Counter5/1, NOT1/1
  Counter1/1 -> Switch3/1
  Switch3/1 -> Switch/1
  NOT1/1 -> Switch3/2
  Delay/1 -> Product1/2
  Delay1/1 -> Product/2
  Constant/1 -> Product/1
  OR/1 -> Switch/2
  NOT2/1 -> OR/2
  NOT3/1 -> OR1/2
  OR1/1 -> Switch1/2  "Check special"
  Constant1/1 -> Product1/1
  Constant2/1 -> Add/1
  Add/1 -> Switch2/1
  Counter3/2 -> S-R Flip-Flop/1
  S-R Flip-Flop/2 -> AND/2
  AND/1 -> Switch2/2  "supercheck"
  Counter3/1 -> Switch1/3
  Counter4/1 -> Subtract/1  "reout"
  Constant3/1 -> Subtract/2
  Subtract/1 -> Switch2/3
  Compare To Constant5/1 -> HCEV1/2
  Compare To Constant4/1 -> HCEV1/1
  HCEV2/1 -> HCEV SOC/1
  Constant4/1 -> HCEV2/1
  HCEV1 Up/1 -> HCEV2/2
  AND1/1 -> Counter3/1, NOT3/1  "supercheck"
  Bilat 2 Discharge/1 -> AND1/1
  Compare To Zero2/1 -> AND1/2
  Subtract5/1 -> Compare To Zero2/1
  Product1/1 -> Switch5/1, Subtract5/1
  Bilateral Partition/1 -> Subtract5/2
  Constant5/1 -> Switch4/3
  Product/1 -> Switch4/1
  EV1/1 -> Switch4/2, EV1 Stat/1
  Switch4/1 -> EV1 SOC/1
  EV2/1 -> Switch5/2, EV2 Stat/1
  Constant6/1 -> Switch5/3
  Switch5/1 -> EV2 SOC/1

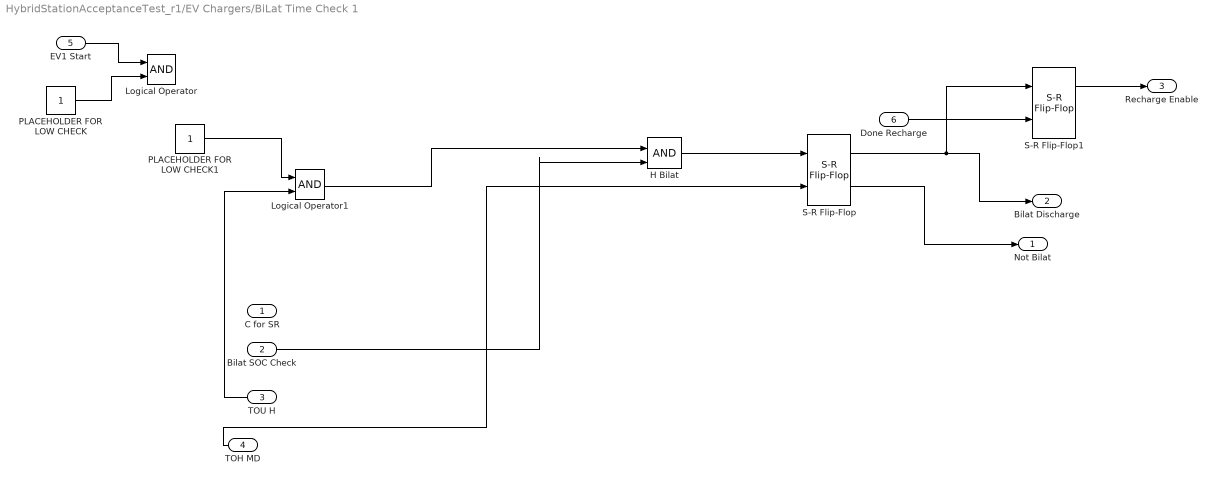
== system HybridStationAcceptanceTest_r1/EV Chargers/BiLat Time Check 1 ==
  C for SR : Inport
  Bilat SOC Check : Inport  Port=2
  TOU H : Inport  Port=3
  TOH MD : Inport  Port=4
  EV1 Start : Inport  Port=5
  Done Recharge : Inport  Port=6
  H Bilat : Logic  IconShape=distinctive  AllPortsSameDT=off  OutDataTypeStr=boolean
  Logical Operator : Logic  AllPortsSameDT=off  OutDataTypeStr=boolean
  Logical Operator1 : Logic  AllPortsSameDT=off  OutDataTypeStr=boolean
  PLACEHOLDER FOR LOW CHECK : Constant
  PLACEHOLDER FOR LOW CHECK1 : Constant
  S-R Flip-Flop : simulink_extras/Flip Flops/S-R Flip-Flop  initial_condition=0
  S-R Flip-Flop1 : simulink_extras/Flip Flops/S-R Flip-Flop  initial_condition=0
  Not Bilat : Outport
  Bilat Discharge : Outport  Port=2
  Recharge Enable : Outport  Port=3
  wires:
  TOH MD/1 -> S-R Flip-Flop/2
  Logical Operator1/1 -> H Bilat/1
  PLACEHOLDER FOR LOW CHECK1/1 -> Logical Operator1/1
  H Bilat/1 -> S-R Flip-Flop/1
  S-R Flip-Flop/1 -> S-R Flip-Flop1/1, Bilat Discharge/1
  S-R Flip-Flop/2 -> Not Bilat/1
  Bilat SOC Check/1 -> H Bilat/2
  TOU H/1 -> Logical Operator1/2
  PLACEHOLDER FOR LOW CHECK/1 -> Logical Operator/2
  EV1 Start/1 -> Logical Operator/1
  S-R Flip-Flop1/1 -> Recharge Enable/1
  Done Recharge/1 -> S-R Flip-Flop1/2

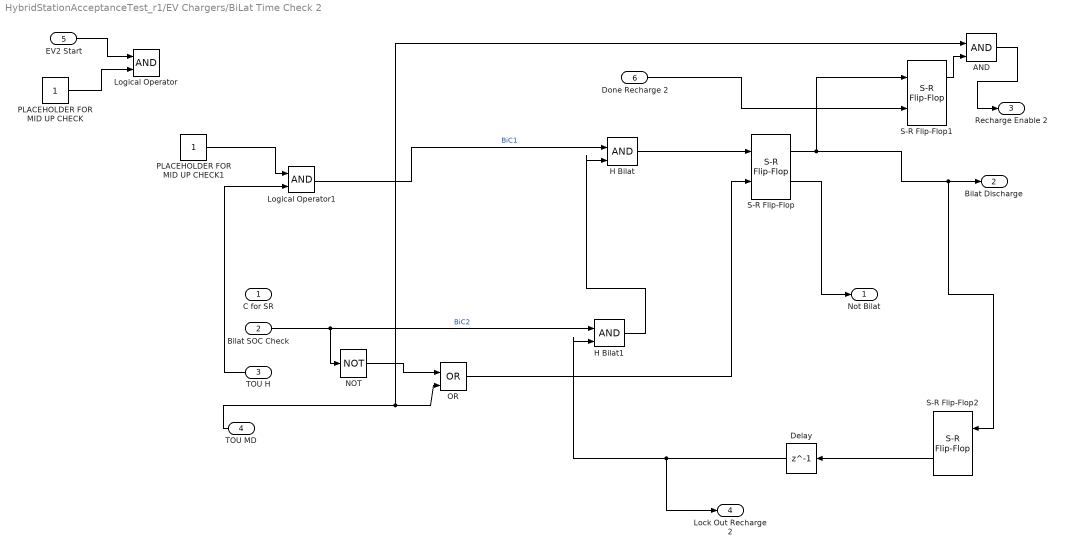
== system HybridStationAcceptanceTest_r1/EV Chargers/BiLat Time Check 2 ==
  C for SR : Inport
  Bilat SOC Check : Inport  Port=2
  TOU H : Inport  Port=3
  TOU MD : Inport  Port=4
  EV2 Start : Inport  Port=5
  Done Recharge 2 : Inport  Port=6
  AND : Logic  IconShape=distinctive  AllPortsSameDT=off  OutDataTypeStr=boolean
  Delay : Delay  DelayLength=1  InitialCondition=0
  H Bilat : Logic  IconShape=distinctive  AllPortsSameDT=off  OutDataTypeStr=boolean
  H Bilat1 : Logic  IconShape=distinctive  AllPortsSameDT=off  OutDataTypeStr=boolean
  Logical Operator : Logic  AllPortsSameDT=off  OutDataTypeStr=boolean
  Logical Operator1 : Logic  AllPortsSameDT=off  OutDataTypeStr=boolean
  NOT : Logic  Operator=NOT  IconShape=distinctive  AllPortsSameDT=off  OutDataTypeStr=boolean
  OR : Logic  Operator=OR  IconShape=distinctive  AllPortsSameDT=off  OutDataTypeStr=boolean
  PLACEHOLDER FOR MID UP CHECK : Constant
  PLACEHOLDER FOR MID UP CHECK1 : Constant
  S-R Flip-Flop : simulink_extras/Flip Flops/S-R Flip-Flop  initial_condition=0
  S-R Flip-Flop1 : simulink_extras/Flip Flops/S-R Flip-Flop  initial_condition=0
  S-R Flip-Flop2 : simulink_extras/Flip Flops/S-R Flip-Flop  initial_condition=0
  Not Bilat : Outport
  Bilat Discharge : Outport  Port=2
  Recharge Enable 2 : Outport  Port=3
  Lock Out Recharge 2 : Outport  Port=4
  wires:
  Logical Operator1/1 -> H Bilat/1  "BiC1"
  PLACEHOLDER FOR MID UP CHECK1/1 -> Logical Operator1/1
  S-R Flip-Flop/1 -> S-R Flip-Flop1/1, S-R Flip-Flop2/1, Bilat Discharge/1
  H Bilat/1 -> S-R Flip-Flop/1
  S-R Flip-Flop/2 -> Not Bilat/1
  Bilat SOC Check/1 -> H Bilat1/1, NOT/1  "BiC2"
  TOU H/1 -> Logical Operator1/2
  EV2 Start/1 -> Logical Operator/1
  PLACEHOLDER FOR MID UP CHECK/1 -> Logical Operator/2
  TOU MD/1 -> AND/1, OR/2
  Done Recharge 2/1 -> S-R Flip-Flop1/2
  AND/1 -> Recharge Enable 2/1
  OR/1 -> S-R Flip-Flop/2
  NOT/1 -> OR/1
  H Bilat1/1 -> H Bilat/2
  S-R Flip-Flop2/2 -> Delay/1
  Delay/1 -> Lock Out Recharge 2/1, H Bilat1/2
  S-R Flip-Flop1/1 -> AND/2

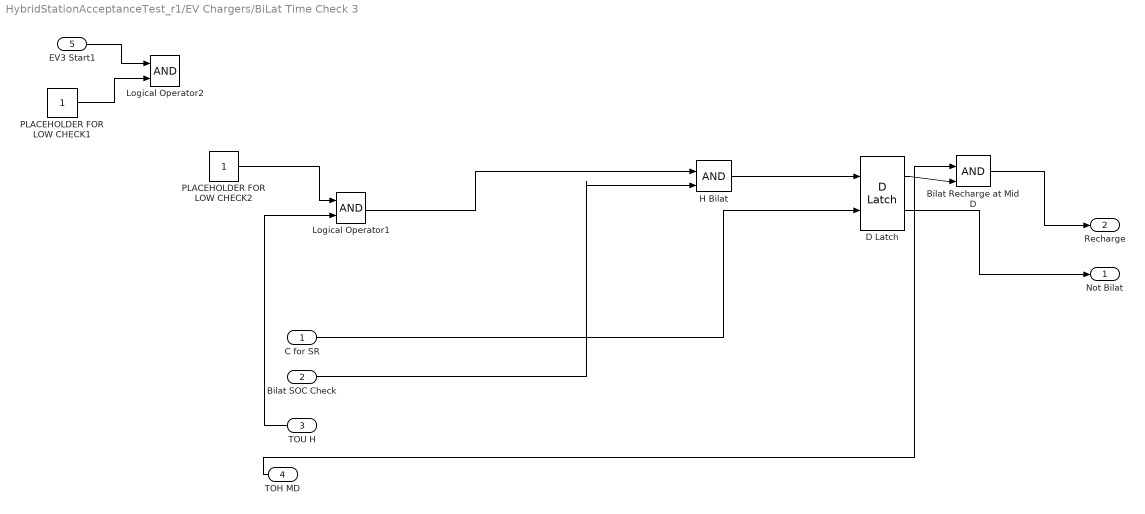
== system HybridStationAcceptanceTest_r1/EV Chargers/BiLat Time Check 3 ==
  C for SR : Inport
  Bilat SOC Check : Inport  Port=2
  TOU H : Inport  Port=3
  TOH MD : Inport  Port=4
  EV3 Start1 : Inport  Port=5
  Bilat Recharge at Mid D : Logic  IconShape=distinctive  AllPortsSameDT=off  OutDataTypeStr=boolean
  D Latch : simulink_extras/Flip Flops/D Latch
  H Bilat : Logic  IconShape=distinctive  AllPortsSameDT=off  OutDataTypeStr=boolean
  Logical Operator1 : Logic  AllPortsSameDT=off  OutDataTypeStr=boolean
  Logical Operator2 : Logic  AllPortsSameDT=off  OutDataTypeStr=boolean
  PLACEHOLDER FOR LOW CHECK1 : Constant
  PLACEHOLDER FOR LOW CHECK2 : Constant
  Not Bilat : Outport
  Recharge : Outport  Port=2
  wires:
  TOH MD/1 -> Bilat Recharge at Mid D/1
  Logical Operator1/1 -> H Bilat/1
  PLACEHOLDER FOR LOW CHECK2/1 -> Logical Operator1/1
  Bilat Recharge at Mid D/1 -> Recharge/1
  H Bilat/1 -> D Latch/1
  D Latch/1 -> Bilat Recharge at Mid D/2
  D Latch/2 -> Not Bilat/1
  C for SR/1 -> D Latch/2
  Bilat SOC Check/1 -> H Bilat/2
  TOU H/1 -> Logical Operator1/2
  EV3 Start1/1 -> Logical Operator2/1
  PLACEHOLDER FOR LOW CHECK1/1 -> Logical Operator2/2

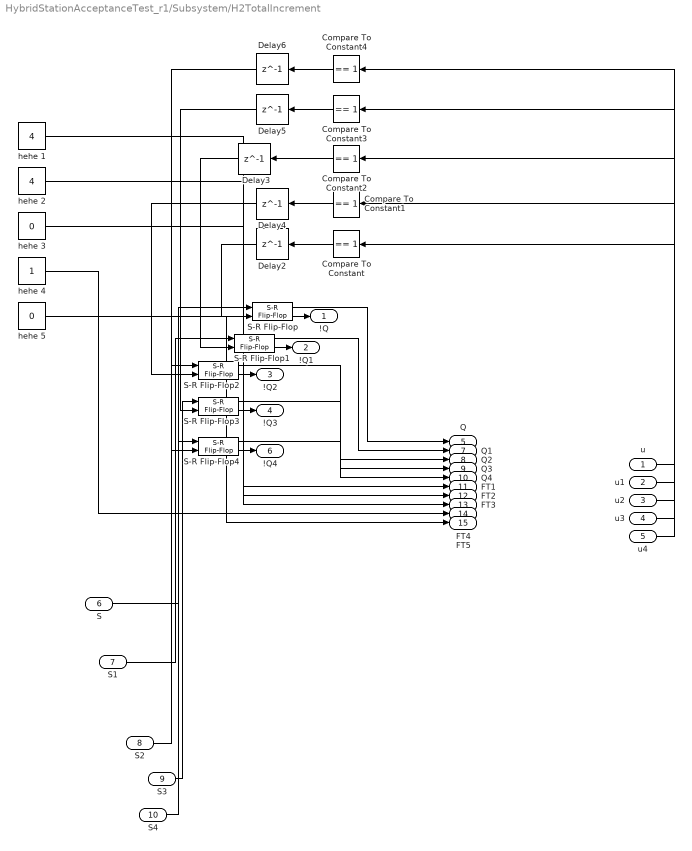
== system HybridStationAcceptanceTest_r1/Subsystem/H2TotalIncrement ==
  u : Inport
  u1 : Inport  Port=2
  u2 : Inport  Port=3
  u3 : Inport  Port=4
  u4 : Inport  Port=5
  S : Inport  Port=6
  S1 : Inport  Port=7
  S2 : Inport  Port=8
  S3 : Inport  Port=9
  S4 : Inport  Port=10
  Compare To Constant{,1..4} (5 alike) : simulink/Logic and Bit Operations/Compare To Constant  relop===  const=1  OutDataTypeStr=boolean
  Delay{2..6} (5 alike) : Delay  DelayLength=1  InitialCondition=0
  S-R Flip-Flop{,1..4} (5 alike) : simulink_extras/Flip Flops/S-R Flip-Flop  initial_condition=0
  hehe 1 : Constant  Value=4
  hehe 2 : Constant  Value=4
  hehe 3 : Constant  Value=0
  hehe 4 : Constant
  hehe 5 : Constant  Value=0
  !Q : Outport
  !Q1 : Outport  Port=2
  !Q2 : Outport  Port=3
  !Q3 : Outport  Port=4
  Q : Outport  Port=5
  !Q4 : Outport  Port=6
  Q1 : Outport  Port=7
  Q2 : Outport  Port=8
  Q3 : Outport  Port=9
  Q4 : Outport  Port=10
  FT1 : Outport  Port=11
  FT2 : Outport  Port=12
  FT3 : Outport  Port=13
  FT4 : Outport  Port=14
  FT5 : Outport  Port=15
  wires:
  u4/1 -> Compare To Constant4/1
  S-R Flip-Flop/2 -> !Q/1
  Delay2/1 -> S-R Flip-Flop/2
  Delay4/1 -> S-R Flip-Flop2/2
  hehe 3/1 -> FT3/1
  S3/1 -> S-R Flip-Flop3/1
  hehe 4/1 -> FT4/1
  u3/1 -> Compare To Constant3/1
  Delay6/1 -> S-R Flip-Flop4/2
  Compare To Constant4/1 -> Delay6/1
  Compare To Constant1/1 -> Delay4/1
  Compare To Constant3/1 -> Delay5/1
  Compare To Constant2/1 -> Delay3/1
  Compare To Constant/1 -> Delay2/1
  Delay3/1 -> S-R Flip-Flop1/2
  S-R Flip-Flop1/2 -> !Q1/1
  Delay5/1 -> S-R Flip-Flop3/2
  S-R Flip-Flop/1 -> Q/1
  S-R Flip-Flop4/1 -> Q4/1
  hehe 5/1 -> FT5/1
  S-R Flip-Flop1/1 -> Q1/1
  S4/1 -> S-R Flip-Flop4/1
  u/1 -> Compare To Constant/1
  S-R Flip-Flop3/1 -> Q3/1
  u1/1 -> Compare To Constant2/1
  S-R Flip-Flop2/2 -> !Q2/1
  S1/1 -> S-R Flip-Flop1/1
  S-R Flip-Flop2/1 -> Q2/1
  S/1 -> S-R Flip-Flop/1
  hehe 1/1 -> FT1/1
  u2/1 -> Compare To Constant1/1
  hehe 2/1 -> FT2/1
  S2/1 -> S-R Flip-Flop2/1
  S-R Flip-Flop4/2 -> !Q4/1
  S-R Flip-Flop3/2 -> !Q3/1

== matlab function HybridStationAcceptanceTest_r1/Total Resource Counter ==
  data: Hydrol input; KHWUSED output; Electrol input; Flyin input; Flyout input; Carin input; Carout input; KWHOUT output; Condenser input
function [KHWUSED, KWHOUT]= fcn(Hydrol, Electrol, Flyin, Flyout, Carin, Carout, Condenser)

KHWUSED = Hydrol + Flyin + Carin + Condenser;

KWHOUT = Electrol + Flyout + Carout;

KWHOUT = 0;
KHWUSED = 0;

== matlab function HybridStationAcceptanceTest_r1/Flywheel/MATLAB Function ==
  data: y output; Charge input; Discharge input
function y = fcn(Charge, Discharge)

y = 0;

== matlab function HybridStationAcceptanceTest_r1/Flywheel/MATLAB Function1 ==
  data: TOU input; SOC1 output; PowIn output; PowOut output
function [SOC1, PowIn, PowOut]= fcn(TOU)

persistent SOC
if isempty(SOC)
    SOC = 0;
end
maxSOC = 100;
if TOU == 0 && SOC <100
    totalTime = 2.5;
    % MaxSOC = 100;
    tic;

    while toc <= totalTime
        SOC = (toc / totalTime) * maxSOC;
    end
elseif TOU == 4 && SOC > 0
    totalTime = 2.5;
    % MaxSOC = 100;
    tic;

    while toc <= totalTime
        SOC = 100 - (toc / totalTime) * maxSOC;
    end
else
    SOC = SOC;
end

SOC1 = SOC;
PowIn = 0;
PowOut = 0;
% % 
% %     % Set the total time for the timer (in seconds)
% % totalTime = 2.5;
% % 
% % % Set the maximum value for the timer
% % maxValue = 100;
% % 
% % % Initialize the timer
% % tic;
% % 
% % % Loop until the specified duration is reached
% % while toc <= totalTime
% %     % Calculate the current value of the timer (linear interpolation)
% %     currentValue = (toc / totalTime) * maxValue;
% % 
% %     % Display the current value
% %     fprintf('Current timer value: %.2f\n', currentValue);
% % 
% %     % Pause for a short duration to control the loop speed
% %     pause(0.1); % Adjust as needed
% % end
% %

== matlab function HybridStationAcceptanceTest_r1/Subsystem/MATLAB Function ==
  data: FCEVIn input; FCEVPres output
function FCEVPres = fcn(FCEVIn)
Counter = 0;
if FCEVIn == 1
    while Counter < 20
        FCEVPres = 1;
        Counter = Counter + 1
    end
    FCEVPres = 0;
end
FCEVPres =0;

== matlab function HybridStationAcceptanceTest_r1/MATLAB Function1 ==
  data: tou input; on_peak output; off_peak output; mid_peak_lo output; mid_peak_hi output; null output
function [on_peak, off_peak, mid_peak_lo, mid_peak_hi, null] = tou_translate(tou)

if tou == 0
    on_peak = logical(false);
    off_peak = logical(false);
    mid_peak_lo = logical(false);
    mid_peak_hi = logical(false);
    null = logical(true);
elseif tou == 1
    on_peak = logical(false);
    off_peak = logical(true);
    mid_peak_lo = logical(false);
    mid_peak_hi = logical(false);
    null = logical(false);
elseif tou == 2
    on_peak = logical(false);
    off_peak = logical(false);
    mid_peak_lo = logical(true);
    mid_peak_hi = logical(false);
    null = logical(false);
elseif tou == 3
    on_peak = logical(false);
    off_peak = logical(false);
    mid_peak_lo = logical(false);
    mid_peak_hi = logical(true);
    null = logical(false);
elseif tou == 4
    on_peak = logical(true);
    off_peak = logical(false);
    mid_peak_lo = logical(false);
    mid_peak_hi = logical(false);
    null = logical(false);
else
    on_peak = logical(false);
    off_peak = logical(false);
    mid_peak_lo = logical(false);
    mid_peak_hi = logical(false);
    null = logical(true);
end

end

== matlab function HybridStationAcceptanceTest_r1/MATLAB Function ==
  data: clock input; time output; smplTime input; dt output; tou output; simTime input; simLength input; szn input; days input; tou_int output
function [time, dt, tou, tou_int] = fcn(clock, smplTime, simTime, simLength, szn, days)
    % Adjusted simulation time to span over 'days' days
    % First, calculate the total simulation time in hours for the given number of days
    totalSimHours = simLength * days;
    
    % Convert clock (in seconds) to actual simulation time (in hours)
    % Instead of scaling the entire simulation to fit within a single day,
    % scale it based on the total simulation hours specified by 'days'
    scalingFactor = totalSimHours / (simTime / 3600);
    scaledTime = clock / 3600 * scalingFactor; % Convert clock to hours and scale based on totalSimHours
    
    tou = "null";
    tou_int = 0;

    % Outputs
    time = scaledTime; % The scaled simulation time in hours, adjusted for multiple days
    dt = (smplTime / simTime) * scaledTime; % The timestep in hours

    % Determine the time of use (TOU) state based on the scaled simulation time
    % For TOU calculations, use mod(time, 24) to determine the time of day for TOU state decisions
    currentTimeOfDay = mod(time, 24);

    % Assuming the 'hrs' variable represents an hour in the context of currentTimeOfDay
    hrs = 1; % 1 hour in terms of scaled simulation time

    % Update TOU state checks to use currentTimeOfDay for daily cycle logic
    if szn == 0
        if (currentTimeOfDay >= 0*hrs && currentTimeOfDay <= 7*hrs) || (currentTimeOfDay > 19*hrs && currentTimeOfDay <= 24*hrs)
            tou = "off_peak";
            tou_int = 1; % off peak
        elseif (currentTimeOfDay > 7*hrs && currentTimeOfDay <= 11*hrs)
            tou = "mid_peak_hi";
            tou_int = 3; % mid peak hi
        elseif (currentTimeOfDay > 11*hrs && currentTimeOfDay <= 17*hrs)
            tou = "on_peak";
            tou_int = 4; % on peak
        elseif (currentTimeOfDay > 17*hrs && currentTimeOfDay <= 19*hrs)
            tou = "mid_peak_lo";
            tou_int = 2; % mid peak lo
        else
            tou = "null";
            tou_int = 0; % null/error
        end
    elseif szn == 1
        if (currentTimeOfDay >= 0*hrs && currentTimeOfDay <= 7*hrs) || (currentTimeOfDay > 19*hrs && currentTimeOfDay <= 24*hrs)
            tou = "off_peak";
            tou_int = 1; % off peak
        elseif (currentTimeOfDay > 7*hrs && currentTimeOfDay <= 11*hrs)
            tou = "on_peak";
            tou_int = 4; % on peak
        elseif (currentTimeOfDay > 11*hrs && currentTimeOfDay <= 17*hrs)
            tou = "mid_peak_lo";
            tou_int = 2; % mid peak lo
        elseif (currentTimeOfDay > 17*hrs && currentTimeOfDay <= 19*hrs)
            tou = "on_peak";
            tou_int = 4; % on peak
        else
            tou = "null";
        end
    end 
end

== matlab function HybridStationAcceptanceTest_r1/Subsystem/HighPressure ==
  data: H70exp input; Pressurize output; FCEVCheck input; PresIn input; H70Tank output; CurH70 output; counter1 output; counter2 output; condenserOn output
function [Pressurize,H70Tank,CurH70,counter1,counter2,condenserOn]= fcn(H70exp,FCEVCheck,PresIn)
persistent H70tot
if isempty(H70tot)
    H70tot = 0;
end
persistent counter
if isempty(counter)
    counter = 0;
end

if H70tot < 4
    Pressurize = 0;
else
    Pressurize = 0;
end

if  FCEVCheck == 1
    H70tot =+ H70exp;
else
     H70tot = H70tot + 0;
     % pause(1);
end
H70Tank = H70tot +5;
if H70exp <= -1
    H70tot;
end


CurH70 = H70exp + 5 + 0.1*counter;

if CurH70 < 10
    counter = counter +1;
    %pause(10);
    pressurize = 1;
    
end
    counter1 = 0.1*counter;
    counter2 = ((counter1-10)/2)+5
    pressurize = 0;
    
 if CurH70 == 10
       condenserOn = 0;
 else
     condenserOn = 1;
 end
    %     Pressurize = 1;
% else 
%     Pressurize = 0;
% end

== matlab function HybridStationAcceptanceTest_r1/Subsystem/Total Usage ==
  data: Time input; H2Out output; idc output; Done1 output; Done2 output; Done3 output; Done4 output; Done5 output; H70Out output; InitOut output; Init input; H2Feedback input; FT1 input; FT2 input; FT3 input; FT4 input; FT5 input; FSOC1 input; FSOC2 input; FSOC3 input; FSOC4 input; FSOC5 input; H70Bar input
function [H2Out,idc,Done1,Done2,Done3,Done4, Done5, H70Out, InitOut] = fcn(Time, Init, H2Feedback, FT1, FT2, FT3, FT4, FT5, FSOC1, FSOC2, FSOC3, FSOC4, FSOC5,H70Bar)
idc = 0;
Done1 = 0;
Done2 = 0;
Done3 = 0;
Done4 = 0;
Done5 = 0;
InitOut = 0;
%H70Bar = 5;
%if Time == 5
%    H70Out = 5
%end
%if Init == 0
%    H70Bar = 5;
%    InitOut = 1;
%else
 %   H70Out = H70Bar;
%end
%InitOut = 1;

if FT1 == true
    H2Out = H2Feedback + (5 - FSOC1);
    H70Bar = H70Bar - (5 - FSOC1);
    %H70Fin = H70Fin -H70Bar
    Done1 = 1;
    %InitOut = 1;
     
elseif FT2 == true
    H2Out = H2Feedback + (5 - FSOC2);
    H70Bar = H70Bar - (5 - FSOC2);
    %H70Fin = H70Fin -H70Bar
    Done2 = 1;
    %InitOut = 1;
elseif FT3 == true
    H2Out = H2Feedback + (5 - FSOC3);
    H70Bar = H70Bar - (5 - FSOC3);
   % H70Fin = H70Fin -H70Bar
    Done3 = 1;
    %InitOut = 1;
elseif FT4 == true
    H2Out = H2Feedback + (5 - FSOC4);
    H70Bar = H70Bar - (5 - FSOC4);
  %  H70Fin = H70Fin -H70Bar
    Done4 = 1;
    %InitOut = 0;
elseif FT5 == true
    H2Out = H2Feedback + (5 - FSOC5);
    H70Bar = H70Bar - (5 - FSOC5);
    %H70Fin = H70Fin -H70Bar
    Done5 = 1;
   % InitOut = 1;
else
    H2Out = (H2Feedback +0);
    
end
H70Out = H70Bar;

== matlab function HybridStationAcceptanceTest_r1/Subsystem/LowPressure ==
  data: presout output; H35exp input; TOU input; elecout1 output; HydrolIn1 output; H35Tank1 output; ElecInHydOut output
function [presout, elecout1, HydrolIn1,H35Tank1, ElecInHydOut]= fcn(H35exp, TOU)
% persistent wait
% if isempty(wait)
%    wait = 0;
% end
% % if isempty(presout)
% %    presout = 0;
% % end
% if callpres == 1
%    presout = 1;
%     % if wait == 0
%    %     % H35 =-
%    %     presout = 1;
%    %     wait = 1;
%    % 
%    %  else
%    %      % pause(1);
%    %      wait = 0;
%    %      presout = 0;
%    % end
% else
%     presout = 0;
% end
presout = 0;

persistent elecout
if isempty(elecout)
    elecout = 0;
end

persistent HydrolIn
if isempty(HydrolIn)
    HydrolIn = 0;
end

persistent H35Tank
if isempty(H35Tank)
    H35Tank = 0;
end

% if H35Tank > 0
    H35Tank = HydrolIn - H35exp - elecout + 5

% else
%     H35Tank = HydrolIn - H35exp - elecout

if H35Tank < 5 && TOU == 1 || H35Tank < 7 && TOU == 3 || H35Tank < 9 && TOU == 4 || H35Tank < 7 && TOU == 2
%if h tank < 5 AND TOU = off peak || h tank < 7 AND tou = mid (up) high ||
%h tank < 9 AND tou = on peak || h tank < 7 AND tou = mid (down) low
    HydrolIn = HydrolIn + 1;
    elecout = elecout;
    ElecInHydOut = 1;
else 
    elecout = elecout +1;
    HydrolIn = HydrolIn;
    ElecInHydOut = 0;
    TOU;

    
end
elecout1 = elecout;
HydrolIn1 = HydrolIn;
H35Tank1 = H35Tank;

== matlab function HybridStationAcceptanceTest_r1/TOU converter ==
  data: Low input; TOU output; MidU input; High input; MD input
function TOU = fcn(Low,MidU,High,MD)

if Low == 1
    TOU = 0;
elseif MidU == 1
    TOU = 1;
elseif High == 1
    TOU = 2;
elseif MD == 1
    TOU = 3;
else
    TOU = 4;
end
